simulink model "SYS5_4"  (R2021b)
settings: Solver=ode4  StartTime=0.0  StopTime=0.1  FixedStep=0.001  RelTol=1e-3
values from neighbouring files (symbols this model uses):
  Jn = 2*Jd    (= 0.000334)    [main.m]
  K = place(A,B,p)    [main.m]
  Kd = place(Sysd.a,Sysd.b,pd)    [main.m]
  Kdnorm1 = 1/yduk(3)    [main.m]
  ke = (Un-R*In)/wn    (= 0.320333333333)    [main.m]
  km = Mn/In    (= 0.228971962617)    [main.m]
  ku = 20    [main.m]
  La = 10^-3 * 58    (= 0.058)    [main.m]
  R = 8.5    [main.m]
settings Model: Creator=Алекс  LastModifiedBy=vkad
settings SolverCC: AlgebraicLoopSolver=TrustRegion
settings DataIOCC: LimitDataPoints=on  SaveFormat=Array  SignalLoggingSaveFormat=ModelDataLogs  ReturnWorkspaceOutputs=off
settings OptimizationCC: ExpressionDepthLimit=2147483647  LifeSpan=inf
settings DebuggingCC: UnderspecifiedInitializationDetection=Classic  MergeDetectMultiDrivingBlocksExec=none  SolverPrmCheckMsg=warning  FcnCallInpInsideContextMsg=warning  StateNameClashWarn=warning  SFUnexpectedBacktrackingDiag=warning  SFNoUnconditionalDefaultTransitionDiag=warning  SFExecutionAtInitializationDiag=none  SFMachineParentedDataDiag=warning  ArithmeticOperatorsInVariantConditions=warning
settings HardwareCC: ProdBitPerPointer=32  ProdBitPerSizeT=32  ProdBitPerPtrDiffT=32  ProdLargestAtomicFloat=None  ProdIntDivRoundTo=Undefined  ProdEndianess=Unspecified  ProdWordSize=32  ProdHWDeviceType=32-bit Generic
settings ModelReferenceCC: PropagateSignalLabelsOutOfModel=off
settings SFSimCC: SimUseLocalCustomCode=off  CustomCodeUndefinedFunction=UseInterfaceOnly
settings RTWCC: RTWUseLocalCustomCode=off
settings CodeAppCC: StateflowObjectComments=on
settings GRTTargetCC: TargetLangStandard=C89/C90 (ANSI)  CombineOutputUpdateFcns=off  GRTInterface=on
settings ConfigComp: CovMetricSettings=dw  CovSaveCumulativeToWorkspaceVar=on  CovSaveSingleToWorkspaceVar=on  CovExternalEMLEnable=off  CovSFcnEnable=off

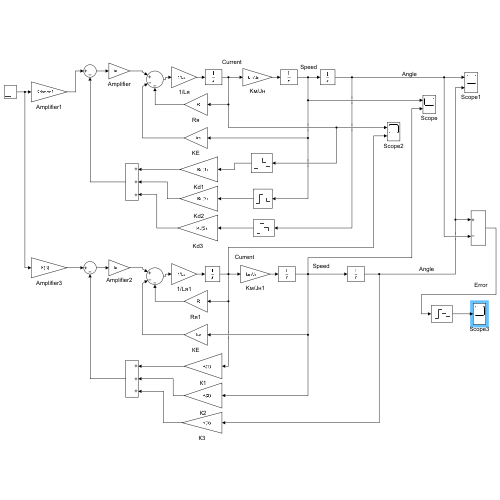
[thumbnail: Simulink's stored preview of the top-level diagram]
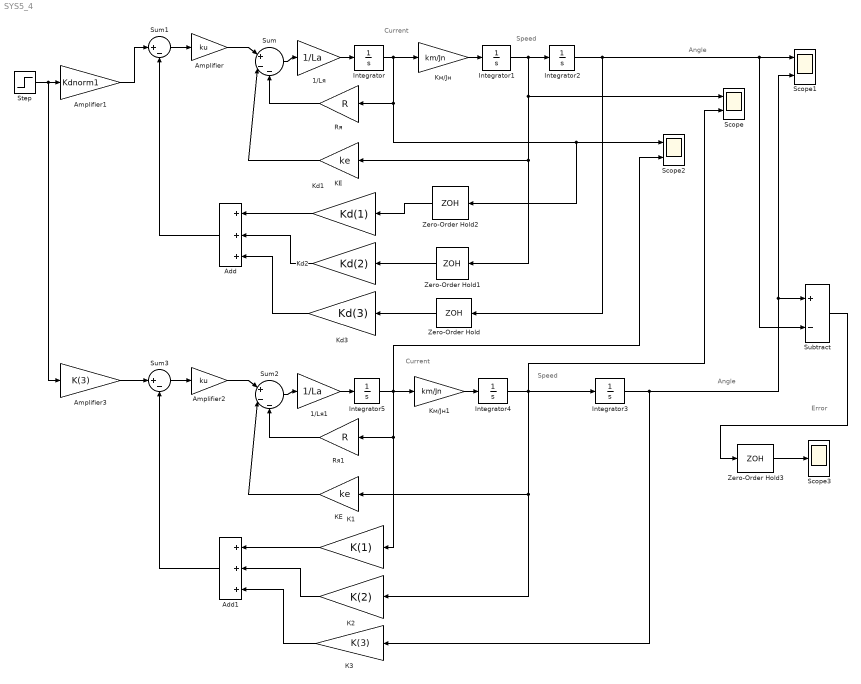
== system SYS5_4 ==
  note: Speed
  note: Angle
  note: Angle
  note: Error
  note: Current
  note: Current
  note: Speed
  1/Lя : Gain  Gain=1/La
  1/Lя1 : Gain  Gain=1/La
  Add : Sum  Inputs=+++
  Add1 : Sum  Inputs=+++
  Amplifier : Gain  Gain=ku
  Amplifier1 : Gain  Gain=Kdnorm1
  Amplifier2 : Gain  Gain=ku
  Amplifier3 : Gain  Gain=K(3)
  Integrator{,1..5} (6 alike) : Integrator
  KE : Gain  Gain=ke
  Kd1 : Gain  Gain=Kd(1)
  Kd2 : Gain  Gain=Kd(2)
  Kd3 : Gain  Gain=Kd(3)
  Kм/Jн : Gain  Gain=km/Jn
  Kм/Jн1 : Gain  Gain=km/Jn
  Rя : Gain  Gain=R
  Rя1 : Gain  Gain=R
  Scope : Scope  NumInputPorts=2
  Scope1 : Scope  NumInputPorts=2
  Scope2 : Scope  NumInputPorts=2
  Scope3 : Scope
  Step : Step  Time=0  SampleTime=0
  Subtract : Sum  Inputs=+-
  Sum : Sum  Inputs=|+--
  Sum1 : Sum  Inputs=|+-
  Sum2 : Sum  Inputs=|+--
  Sum3 : Sum  Inputs=|+-
  Zero-Order Hold{,1..3} (4 alike) : ZeroOrderHold  SampleTime=0.001
  К1 : Gain  Gain=K(1)
  К2 : Gain  Gain=K(2)
  К3 : Gain  Gain=K(3)
  КЕ : Gain  Gain=ke
  wires:
  Sum/1 -> 1/Lя/1
  Integrator1/1 -> Integrator2/1, Zero-Order Hold1/1, KE/1, Scope/1
  Integrator2/1 -> Subtract/2, Scope1/1, Zero-Order Hold/1
  1/Lя/1 -> Integrator/1
  Rя/1 -> Sum/3
  KE/1 -> Sum/2
  Sum1/1 -> Amplifier/1
  Amplifier/1 -> Sum/1
  Step/1 -> Amplifier3/1, Amplifier1/1
  Kd1/1 -> Add/1
  Kd2/1 -> Add/2
  Kd3/1 -> Add/3
  Sum2/1 -> 1/Lя1/1
  Kм/Jн1/1 -> Integrator4/1
  Integrator5/1 -> Scope2/2, Kм/Jн1/1, Rя1/1, К1/1
  1/Lя1/1 -> Integrator5/1
  Rя1/1 -> Sum2/3
  КЕ/1 -> Sum2/2
  Sum3/1 -> Amplifier2/1
  Amplifier2/1 -> Sum2/1
  К1/1 -> Add1/1
  К2/1 -> Add1/2
  К3/1 -> Add1/3
  Kм/Jн/1 -> Integrator1/1
  Integrator3/1 -> К3/1, Subtract/1, Scope1/2
  Integrator4/1 -> Scope/2, К2/1, КЕ/1, Integrator3/1
  Zero-Order Hold/1 -> Kd3/1
  Zero-Order Hold1/1 -> Kd2/1
  Zero-Order Hold2/1 -> Kd1/1
  Integrator/1 -> Rя/1, Zero-Order Hold2/1, Scope2/1, Kм/Jн/1
  Amplifier3/1 -> Sum3/1
  Amplifier1/1 -> Sum1/1
  Add/1 -> Sum1/2
  Add1/1 -> Sum3/2
  Subtract/1 -> Zero-Order Hold3/1
  Zero-Order Hold3/1 -> Scope3/1
